simulink model "Microwave2014b"  (R2014b)
settings: Solver=ode45  StartTime=0.0  StopTime=20  RelTol=1e-3
libraries: simulink x1
settings Model: CovSFcnEnable=on  Creator=bourbouh  LastModifiedBy=hamza
settings DataIOCC: SaveFormat=Structure
settings DebuggingCC: SolverPrmCheckMsg=none  FrameProcessingCompatibilityMsg=error

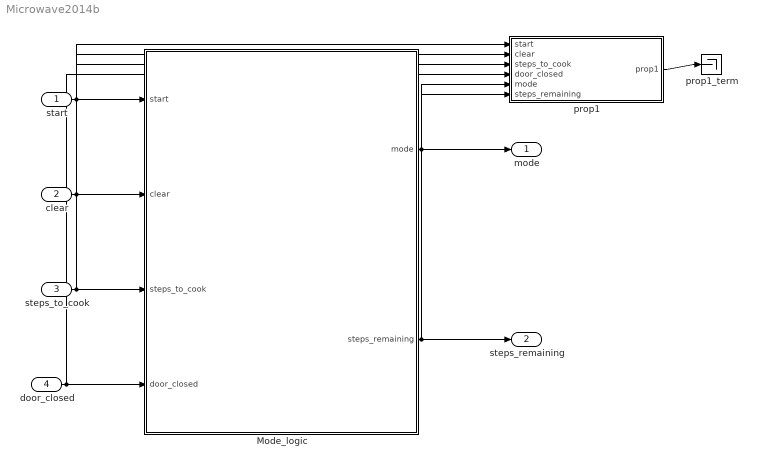
== system Microwave2014b ==
  start : Inport
  clear : Inport  Port=2
  steps_to_cook : Inport  Port=3
  door_closed : Inport  Port=4
  Mode_logic : Stateflow chart  TreatAsAtomicUnit=on
      settings: PermitHierarchicalResolution=ParametersOnly
  prop1 : Subsystem  TreatAsAtomicUnit=on  mask(Observer){AnnotationType=ensures, ObserverType=[]}
      mask prompts: AnnotationType "Type of annotation (pre/post...)"; ObserverType "Observer type"
      mask help:
      | Set an observer for the system.
      | The annotation type parameter sets the type of observer:
      | - requires : pre-condition
      | - ensures : post-condition
      | - assert : an assertion
      | - observer : the observer computes a special type of properties
      mask TypeOptions AnnotationType: ensures | requires | assert | observer
      mask Callback AnnotationType:
      | paramStr = get_param(gcb, 'MaskValues');
      | if strcmp(paramStr{1}(1),'o')
      | set_param(gcb,'MaskVisibilities',{'on';'on'});
      | paramStr{2} = 'ellipsoid';
      | set_param(gcb,'MaskValues',paramStr);
      | else
      | set_param(gcb,'MaskVisibilities',{'on';'off'});
      | end
      | clear paramStr;
      mask Callback ObserverType:
      | paramStr = get_param(gcb, 'MaskValues');
      | if strcmp(paramStr{1}(1),'o')
      | set_param(gcb,'MaskVisibilities',{'on';'on'});
      | paramStr{2} = 'ellipsoid';
      | set_param(gcb,'MaskValues',paramStr);
      | else
      | set_param(gcb,'MaskVisibilities',{'on';'off'});
      | end
      | clear paramStr;
      mask Display:
      | color('black')
      | text(0.5, 0.5, ['Property: ''' get_param(gcb,'name') ''''], 'horizontalAlignment', 'center');
      | text(0.99, 0.03, '{\bf\fontsize{12}SAFE}', 'hor', 'right', 'ver', 'bottom', 'texmode', 'on');
  prop1_term : Terminator
  mode : Outport
  steps_remaining : Outport  Port=2
  wires:
  start/1 -> Mode_logic/1(start), prop1/1(start)
  door_closed/1 -> Mode_logic/4(door_closed), prop1/4(door_closed)
  steps_to_cook/1 -> Mode_logic/3(steps_to_cook), prop1/3(steps_to_cook)
  clear/1 -> Mode_logic/2(clear), prop1/2(clear)
  Mode_logic/1(mode) -> mode/1, prop1/5(mode)
  Mode_logic/2(steps_remaining) -> steps_remaining/1, prop1/6(steps_remaining)
  prop1/1(prop1) -> prop1_term/1

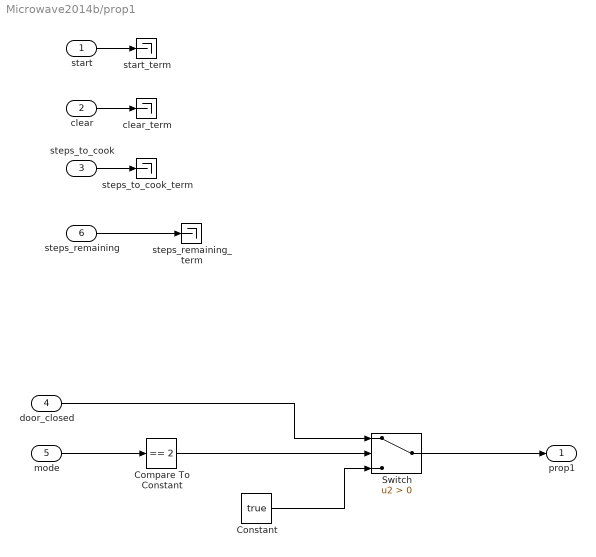
== system Microwave2014b/prop1 ==
  start : Inport
  clear : Inport  Port=2
  steps_to_cook : Inport  Port=3
  door_closed : Inport  Port=4
  mode : Inport  Port=5
  steps_remaining : Inport  Port=6
  Compare To Constant : simulink/Logic and Bit Operations/Compare To Constant  relop===  const=2  OutDataTypeStr=boolean
  Constant : Constant  Value=true
  Switch : Switch  Criteria=u2 > Threshold
  clear_term : Terminator
  start_term : Terminator
  steps_remaining_term : Terminator
  steps_to_cook_term : Terminator
  prop1 : Outport
  wires:
  start/1 -> start_term/1
  clear/1 -> clear_term/1
  steps_to_cook/1 -> steps_to_cook_term/1
  steps_remaining/1 -> steps_remaining_term/1
  door_closed/1 -> Switch/1
  Switch/1 -> prop1/1
  Constant/1 -> Switch/3
  mode/1 -> Compare To Constant/1
  Compare To Constant/1 -> Switch/2

== stateflow chart Microwave2014b/Mode_logic ==
  settings: updateMethod=DISCRETE  sampleTime=1
  state RUNNING
    state COOKING
      entry: mode=2;
    state SUSPENDED
      entry: mode=3;
    COOKING -> COOKING [order 2] : [steps_remaining > 0]
        | /steps_remaining--;
    (default) -> (junction 17)
    (junction 17) -> COOKING [order 1] : [door_closed]
    (junction 17) -> SUSPENDED [order 2]
    SUSPENDED -> COOKING [order 2] : [start && ...
        | door_closed]
    COOKING -> SUSPENDED [order 1] : [clear || ...
        | !door_closed]
  state SETUP
    entry:
    mode=1;
    steps_remaining = steps_to_cook;
  (default) -> SETUP
  SETUP -> (junction 18) : {steps_remaining = steps_to_cook;}
  (junction 18) -> RUNNING : [start && steps_remaining > 0]
  (junction 19) -> SETUP
  RUNNING -> (junction 19) : [steps_remaining <= 0]
  SUSPENDED -> (junction 19) [order 1] : [clear]
  data: start input boolean; clear input boolean; steps_to_cook input uint16; door_closed input boolean; mode output uint8; steps_remaining output uint16 [0..600]
